simulink model "LabPart_2"  (R2023b)
settings: Solver=VariableStepAuto  StartTime=0.0  StopTime=10.0  MaxStep=1e-3  RelTol=1e-3
settings Model: Creator=hp  LastModifiedBy=hp

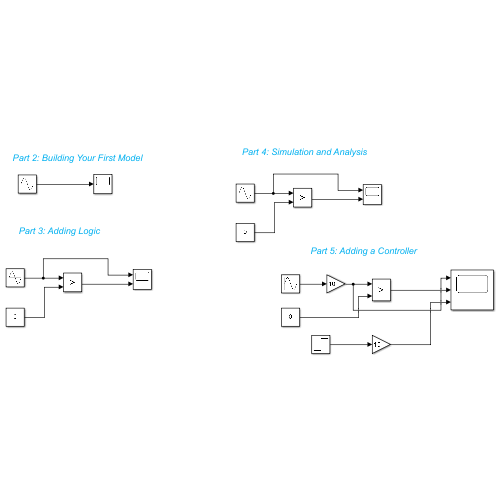
[thumbnail: Simulink's stored preview of the top-level diagram]
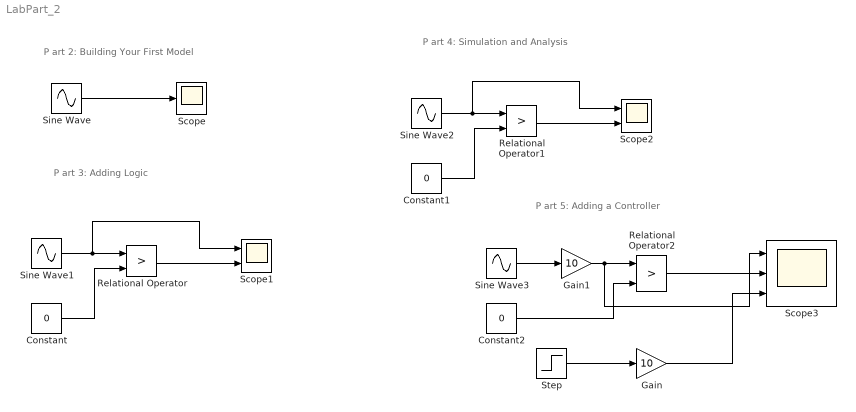
== system LabPart_2 ==
  note: P art 5: Adding a Controller
  note: P art 4: Simulation and Analysis
  note: P art 3: Adding Logic
  note: P art 2: Building Your First Model
  Constant : Constant  Value=0
  Constant1 : Constant  Value=0
  Constant2 : Constant  Value=0
  Gain : Gain  Gain=10
  Gain1 : Gain  Gain=10
  Relational Operator : RelationalOperator  Operator=>  OutDataTypeStr=boolean  RndMeth=Simplest  InputSameDT=off
  Relational Operator1 : RelationalOperator  Operator=>  OutDataTypeStr=boolean  RndMeth=Simplest  InputSameDT=off
  Relational Operator2 : RelationalOperator  Operator=>  OutDataTypeStr=boolean  RndMeth=Simplest  InputSameDT=off
  Scope : Scope
  Scope1 : Scope  NumInputPorts=2
  Scope2 : Scope  NumInputPorts=2
  Scope3 : Scope  NumInputPorts=3
  Sine Wave : Sin  Frequency=2*pi*1  SampleTime=0
  Sine Wave1 : Sin  Frequency=2*pi*1  SampleTime=0
  Sine Wave2 : Sin  Frequency=2*pi*1  Phase=pi  SampleTime=0
  Sine Wave3 : Sin  Frequency=2*pi*1  SampleTime=0
  Step : Step  Time=2  SampleTime=0
  wires:
  Sine Wave/1 -> Scope/1
  Sine Wave1/1 -> Scope1/1, Relational Operator/1
  Constant/1 -> Relational Operator/2
  Relational Operator/1 -> Scope1/2
  Relational Operator1/1 -> Scope2/2
  Constant1/1 -> Relational Operator1/2
  Sine Wave2/1 -> Relational Operator1/1, Scope2/1
  Step/1 -> Gain/1
  Relational Operator2/1 -> Scope3/2
  Gain/1 -> Scope3/3
  Constant2/1 -> Relational Operator2/2
  Gain1/1 -> Scope3/1, Relational Operator2/1
  Sine Wave3/1 -> Gain1/1
